simulink model "ShockAbsorber"  (R2020a)
settings: Solver=VariableStepAuto  StartTime=0.0  StopTime=10.0  MaxStep=0.001  RelTol=1e-3
PostLoadFcn:
  | M1 = 100;
  | K1 = 50;
  | b = 50;
  | a = 2;
  | w0 = 10;
undefined symbols (not defined in the file): M2
settings Model: Creator=Admin  LastModifiedBy=Admin
settings DataIOCC: ExternalInput=[t, F]  LoadExternalInput=on  SaveFormat=Array

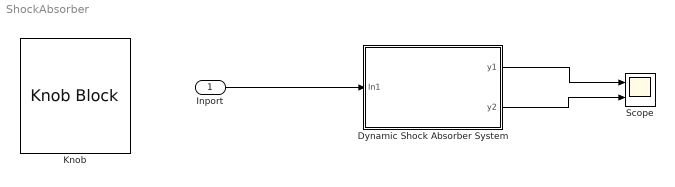
== system ShockAbsorber ==
  Inport : Inport
  Dynamic Shock Absorber System : Subsystem
  Knob : KnobBlock
  Scope : Scope  NumInputPorts=2
  wires:
  Inport/1 -> Dynamic Shock Absorber System/1(In1)
  Dynamic Shock Absorber System/1(y1) -> Scope/1
  Dynamic Shock Absorber System/2(y2) -> Scope/2

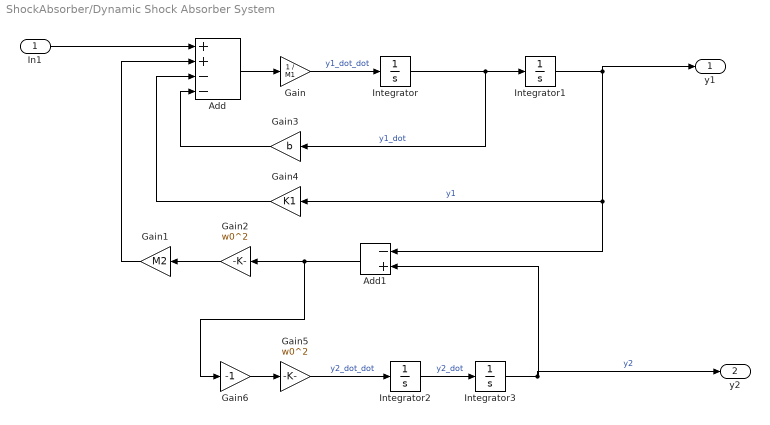
== system ShockAbsorber/Dynamic Shock Absorber System ==
  In1 : Inport
  Add : Sum  Inputs=++--
  Add1 : Sum  Inputs=-+
  Gain : Gain  Gain=1 / M1
  Gain1 : Gain  Gain=M2
  Gain2 : Gain  Gain=w0^2
  Gain3 : Gain  Gain=b
  Gain4 : Gain  Gain=K1
  Gain5 : Gain  Gain=w0^2
  Gain6 : Gain  Gain=-1
  Integrator{,1..3} (4 alike) : Integrator
  y1 : Outport
  y2 : Outport  Port=2
  wires:
  Gain/1 -> Integrator/1  "y1_dot_dot"
  Integrator3/1 -> y2/1, Add1/2  "y2"
  Integrator/1 -> Gain3/1, Integrator1/1  "y1_dot"
  Gain2/1 -> Gain1/1
  Add/1 -> Gain/1
  Gain1/1 -> Add/2
  Integrator2/1 -> Integrator3/1  "y2_dot"
  Integrator1/1 -> y1/1, Add1/1, Gain4/1  "y1"
  Gain3/1 -> Add/4
  Add1/1 -> Gain6/1, Gain2/1
  Gain4/1 -> Add/3
  Gain6/1 -> Gain5/1
  Gain5/1 -> Integrator2/1  "y2_dot_dot"
  In1/1 -> Add/1
